simulink model "Integration_Forward_JFK_Line_Search"  (R2015a)
settings: Solver=ode3  StartTime=0.0  StopTime=T_opt  FixedStep=0.01  MaxStep=0.01  RelTol=1e-3
values from neighbouring files (symbols this model uses):
  H0 = Periodic_Solution(1,4)    [Optimal_Entrainment_shiftworker.m]
  I_update = I    [Optimal_Entrainment_shiftworker.m]
  n0 = Periodic_Solution(1,7)    [Optimal_Entrainment_shiftworker.m]
  Periodic_Solution = Periodic_Solution(1401:end,:)    [Optimal_Entrainment_shiftworker.m]
  shift = 12    [Optimal_Entrainment_shiftworker.m]
  Sleep0 = 0    [Optimal_Entrainment_shiftworker.m]
  Sleep_update = Sleep    [Optimal_Entrainment_shiftworker.m]
  tol = 0.01    [Optimal_Entrainment_shiftworker.m]
  x0 = Periodic_Solution(1,2)    [Optimal_Entrainment_shiftworker.m]
  xc0 = Periodic_Solution(1,3)    [Optimal_Entrainment_shiftworker.m]
settings Model: Creator=wangf7  LastModifiedBy=Jiawei Yin
settings OptimizationCC: ExpressionDepthLimit=2147483647
settings DebuggingCC: AlgebraicLoopMsg=none  ArtificialAlgebraicLoopMsg=none  UnderspecifiedInitializationDetection=Classic  MergeDetectMultiDrivingBlocksExec=none  SolverPrmCheckMsg=warning  StateNameClashWarn=warning

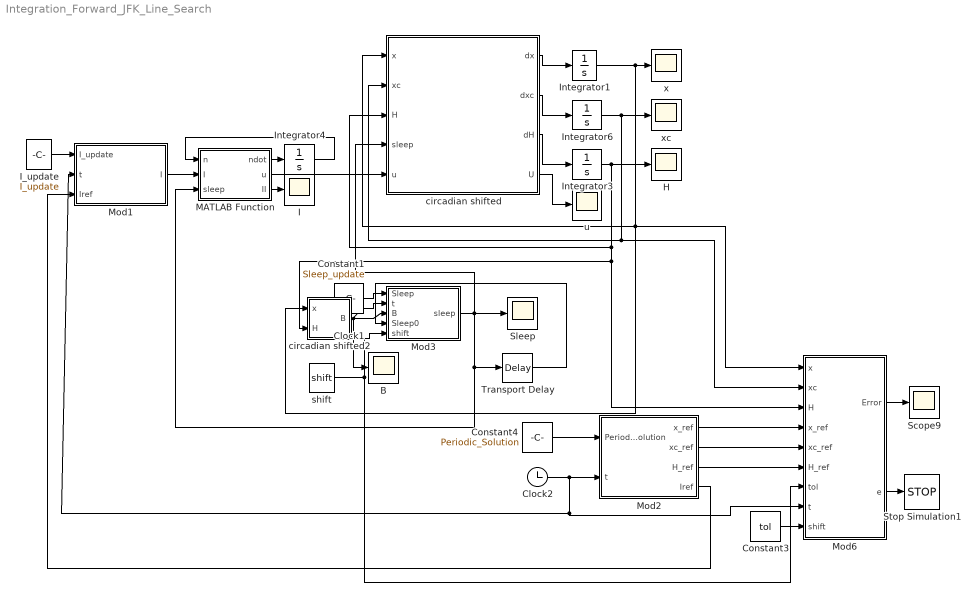
== system Integration_Forward_JFK_Line_Search ==
  B : Scope
      settings: TimeRange=auto  MaxDataPoints=5000  SaveName=B  YMin=0.09109  YMax=0.29109  SampleTime=-1  DataFormat=Array
  Clock1 : Clock
  Clock2 : Clock
  Constant1 : Constant  Value=Sleep_update
  Constant3 : Constant  Value=tol
  Constant4 : Constant  Value=Periodic_Solution
  H : Scope
      settings: TimeRange=auto  MaxDataPoints=5000  SaveName=H_plus  YMin=0.00957  YMax=0.70084  SampleTime=-1  DataFormat=Array
  I : Scope
      settings: TimeRange=auto  MaxDataPoints=5000  SaveName=I_plus  YMin=-10  YMax=10  SampleTime=-1  DataFormat=Array
  I_update : Constant  Value=I_update
  Integrator1 : Integrator  InitialCondition=x0
  Integrator3 : Integrator  InitialCondition=H0
  Integrator4 : Integrator  InitialCondition=n0
  Integrator6 : Integrator  InitialCondition=xc0
  MATLAB Function : MATLAB Function  TreatAsAtomicUnit=on
      settings: PermitHierarchicalResolution=ParametersOnly
  Mod1 : MATLAB Function  TreatAsAtomicUnit=on
      settings: PermitHierarchicalResolution=ParametersOnly
  Mod2 : MATLAB Function  TreatAsAtomicUnit=on
      settings: PermitHierarchicalResolution=ParametersOnly
  Mod3 : MATLAB Function  TreatAsAtomicUnit=on
      settings: PermitHierarchicalResolution=ParametersOnly
  Mod6 : MATLAB Function  TreatAsAtomicUnit=on
      settings: PermitHierarchicalResolution=ParametersOnly
  Scope9 : Scope
      settings: TimeRange=auto  MaxDataPoints=5000  SaveName=Error_plus  YMin=0.06228  YMax=0.08228  SampleTime=-1  DataFormat=Array
  Sleep : Scope
      settings: TimeRange=auto  MaxDataPoints=5000  SaveName=Sleep_plus  YMin=-0.125  YMax=1.125  SampleTime=-1  DataFormat=Array
  Stop Simulation1 : Stop
  Transport Delay : TransportDelay  DelayTime=.01  InitialOutput=Sleep0
  circadian shifted : MATLAB Function  TreatAsAtomicUnit=on
      settings: PermitHierarchicalResolution=ParametersOnly
  circadian shifted2 : MATLAB Function  TreatAsAtomicUnit=on
      settings: PermitHierarchicalResolution=ParametersOnly
  shift : Constant  Value=shift
  u : Scope
      settings: TimeRange=auto  MaxDataPoints=5000  SaveName=u_plus  YMin=0.08613  YMax=0.10613  SampleTime=-1  DataFormat=Array
  x : Scope
      settings: TimeRange=auto  MaxDataPoints=5000  SaveName=x_plus  YMin=-0.81237  YMax=-0.61237  SampleTime=-1  DataFormat=Array
  xc : Scope
      settings: TimeRange=auto  MaxDataPoints=5000  SaveName=xc_plus  YMin=0.62881  YMax=0.82881  SampleTime=-1  DataFormat=Array
  wires:
  circadian shifted/1(dx) -> Integrator1/1
  Integrator1/1 -> circadian shifted2/1(x), Mod6/1(x), circadian shifted/1(x), x/1
  Integrator6/1 -> Mod6/2(xc), circadian shifted/2(xc), xc/1
  Constant4/1 -> Mod2/1(Periodic_Solution)
  Mod6/2(e) -> Stop Simulation1/1
  Mod6/1(Error) -> Scope9/1
  Mod2/3(H_ref) -> Mod6/6(H_ref)
  Constant3/1 -> Mod6/7(tol)
  circadian shifted/2(dxc) -> Integrator6/1
  circadian shifted/3(dH) -> Integrator3/1
  Integrator3/1 -> circadian shifted2/2(H), Mod6/3(H), circadian shifted/3(H), H/1
  Mod2/1(x_ref) -> Mod6/4(x_ref)
  Mod2/2(xc_ref) -> Mod6/5(xc_ref)
  circadian shifted/4(U) -> u/1
  I_update/1 -> Mod1/1(I_update)
  Mod1/1(I) -> MATLAB Function/2(I)
  MATLAB Function/1(ndot) -> Integrator4/1
  Integrator4/1 -> MATLAB Function/1(n)
  MATLAB Function/3(II) -> I/1
  MATLAB Function/2(u) -> circadian shifted/5(u)
  circadian shifted2/1(B) -> Mod3/3(B), B/1
  Mod3/1(sleep) -> MATLAB Function/3(sleep), Transport Delay/1, Sleep/1, circadian shifted/4(sleep)
  Constant1/1 -> Mod3/1(Sleep)
  Clock1/1 -> Mod3/2(t)
  Transport Delay/1 -> Mod3/4(Sleep0)
  Mod2/4(Iref) -> Mod1/3(Iref)
  shift/1 -> Mod6/9(shift), Mod3/5(shift)
  Clock2/1 -> Mod6/8(t), Mod1/2(t), Mod2/2(t)

== matlab function Integration_Forward_JFK_Line_Search/Mod1 ==
  data: I_update input; I output; t input; Iref input
function I  = fcn(I_update,t,Iref)
%#codegen
if t<=I_update(end,1)
    I=interp1q(I_update(:,1),I_update(:,2),t);
else
    I=Iref;
end

== matlab function Integration_Forward_JFK_Line_Search/Mod3 ==
  data: Sleep input; sleep output; t input; B input; Sleep0 input; shift input
function sleep = fcn(Sleep,t,B,Sleep0,shift)
%#codegen
if t<=Sleep(end,1)
    sleep=round(interp1q(Sleep(:,1),Sleep(:,2),t)); 
    if round(sleep)==0 && round(Sleep0)==1
        if B>=0.27
            sleep=1;
        end 
    elseif round(sleep)==1 && round(Sleep0)==0
        if B<0.67
            sleep=0;
        end
    end
    if B>=0.77
        sleep=1;
    elseif B<=0.17
        sleep=0;
    end
else
    sleep=round(Sleep0);
    if B>=0.67
        sleep=1;
    elseif B<=0.17
       sleep=0;
   end
end

if t<shift
    sleep=0;
end

== matlab function Integration_Forward_JFK_Line_Search/MATLAB Function ==
  data: n input; I input; ndot output; u output; sleep input; II output
function [ndot,u,II] = fcn(n,I,sleep)
G=33.75;
alpha0=0.05;
beta=0.0075;
I0=9500;
II=I*(1-sleep);
alpha=alpha0*(I/I0)^0.5;
u=G*alpha*(1-n)*(1-sleep);
ndot=60*[alpha*(1-n)*(1-sleep)-beta*n];

== matlab function Integration_Forward_JFK_Line_Search/circadian shifted ==
  data: x input; xc input; H input; sleep input; u input; dx output; dxc output; dH output; U output
function [ dx,dxc,dH,U] = fcn(x,xc,H,sleep,u)
%#eml

tr=18.2;
td=4.2;

q = 1/3;
taux = 24.2;
k = 0.55;
mu=0.13;
U=u*(1-sleep);
B = u*(1-0.4*x)*(1-0.4*xc)*(1-sleep);

dx = (pi/12)*(xc + B  + mu*(1/3*x + 4/3*x^3 - 256/105*x^7));
dxc = (pi/12)*(q*B *xc - (24/(taux*0.99729))^2*x - k*B*x);
dH = (1-sleep)*(1-H)/tr-(H*sleep)/td;

== matlab function Integration_Forward_JFK_Line_Search/circadian shifted2 ==
  data: x input; H input; B output
function B = fcn(x,H)
%#eml
B=H-0.1333*x;

== matlab function Integration_Forward_JFK_Line_Search/Mod2 ==
  data: Periodic_Solution input; x_ref output; xc_ref output; t input; H_ref output; Iref output
function [x_ref,xc_ref,H_ref,Iref] = fcn(Periodic_Solution,t)
%#codegen
x_ref=interp1q(Periodic_Solution(:,1),Periodic_Solution(:,2),t);
xc_ref=interp1q(Periodic_Solution(:,1),Periodic_Solution(:,3),t);
H_ref=interp1q(Periodic_Solution(:,1),Periodic_Solution(:,4),t);
Iref=interp1q(Periodic_Solution(:,1),Periodic_Solution(:,5),t);

== matlab function Integration_Forward_JFK_Line_Search/Mod6 ==
  data: Error output; x input; xc input; H input; x_ref input; xc_ref input; e output; H_ref input; tol input; t input; shift input
function [Error,e] = fcn(x,xc,H,x_ref,xc_ref,H_ref,tol,t,shift)
%#codegen
Error=(H-H_ref)^2+(x-x_ref)^2+(xc-xc_ref)^2;
e=Error<tol && t>shift;
